simulink model "Model"  (R2021b)
settings: Solver=VariableStepAuto  StartTime=0.0  StopTime=10  RelTol=1e-3
undefined symbols (not defined in the file): A, Am, B, Bm, C, C2, Cm, D, D2, Dm, gamma, gammar, kr, kx, P
settings Model: Creator=Daniel  LastModifiedBy=Daniel

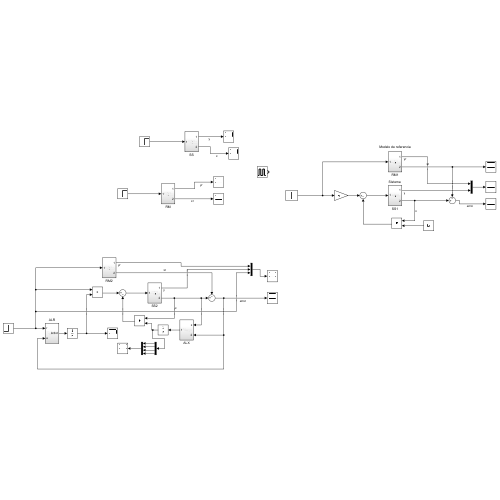
[thumbnail: Simulink's stored preview of the top-level diagram]
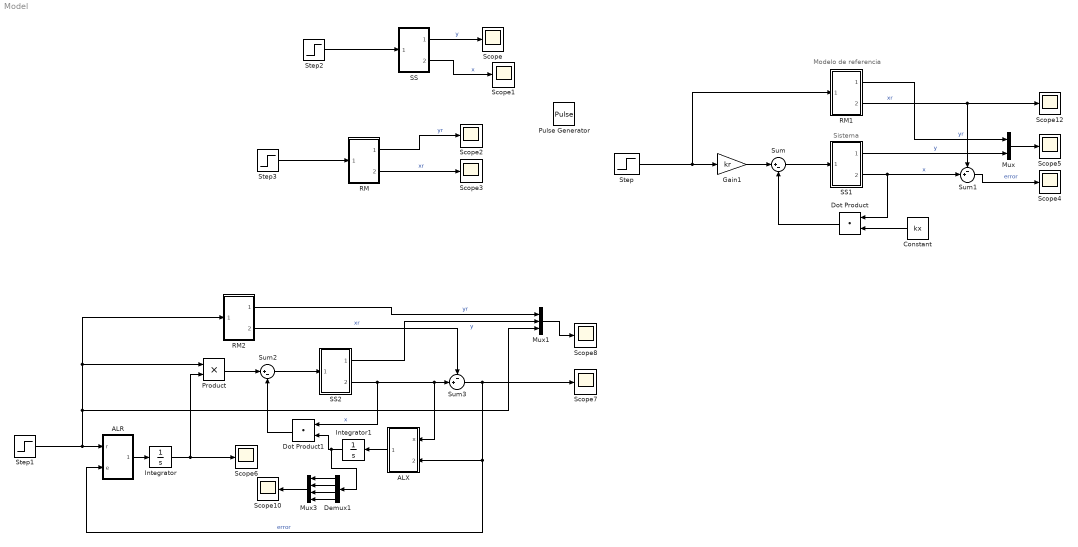
== system Model ==
  note: Sistema
  note: Modelo de referencia
  ALR : Subsystem
  ALX : Subsystem
  Constant : Constant  Value=kx
  Demux1 : Demux
  Dot Product : DotProduct  InputSameDT=on  OutDataTypeStr=Inherit: Inherit via internal rule
  Dot Product1 : DotProduct  InputSameDT=on  OutDataTypeStr=Inherit: Inherit via internal rule
  Gain1 : Gain  Gain=kr
  Integrator : Integrator  InitialCondition=kr
  Integrator1 : Integrator  InitialCondition=[kx]
  Mux : Mux  Inputs=2
  Mux1 : Mux  Inputs=3
  Mux3 : Mux
  Product : Product
  Pulse Generator : DiscretePulseGenerator  PulseType=Time based  Period=5  PulseWidth=50
  RM : Subsystem
  RM1 : Subsystem
  RM2 : Subsystem
  SS : Subsystem
  SS1 : Subsystem
  SS2 : Subsystem
  Scope{,1..8,10,12} (11 alike) : Scope
  Step : Step  Time=0  SampleTime=0
  Step1 : Step  SampleTime=0
  Step2 : Step  SampleTime=0
  Step3 : Step  Time=0  SampleTime=0
  Sum : Sum  Inputs=|+-
  Sum1 : Sum  Inputs=-+|
  Sum2 : Sum  Inputs=|+-
  Sum3 : Sum  Inputs=-+|
  wires:
  Step2/1 -> SS/1(In1)
  SS/1(Out1) -> Scope/1  "y"
  SS/2(Out2) -> Scope1/1  "x"
  Step3/1 -> RM/1(In1)
  RM/1(Out1) -> Scope2/1  "yr"
  RM/2(Out2) -> Scope3/1  "xr"
  SS1/2(Out2) -> Dot Product/1, Sum1/2  "x"
  Sum/1 -> SS1/1(In1)
  RM1/2(Out2) -> Scope12/1, Sum1/1  "xr"
  Dot Product/1 -> Sum/2
  Gain1/1 -> Sum/1
  Step/1 -> Gain1/1, RM1/1(In1)
  Sum1/1 -> Scope4/1  "error"
  Constant/1 -> Dot Product/2
  Sum3/1 -> Scope7/1, ALR/2(e), ALX/2(In2)  "error"
  Product/1 -> Sum2/1
  Dot Product1/1 -> Sum2/2
  RM2/2(Out2) -> Sum3/1  "xr"
  Sum2/1 -> SS2/1(In1)
  SS2/2(Out2) -> ALX/1(x), Sum3/2, Dot Product1/1  "x"
  ALR/1(krdot) -> Integrator/1
  Integrator/1 -> Scope6/1, Product/2
  ALX/1(Out1) -> Integrator1/1
  Integrator1/1 -> Demux1/1, Dot Product1/2
  Mux/1 -> Scope5/1
  RM1/1(Out1) -> Mux/1  "yr"
  SS1/1(Out1) -> Mux/2  "y"
  Step1/1 -> RM2/1(In1), Product/1, Mux1/3, ALR/1(r)
  RM2/1(Out1) -> Mux1/1  "yr"
  SS2/1(Out1) -> Mux1/2  "y"
  Mux1/1 -> Scope8/1
  Mux3/1 -> Scope10/1
  Demux1/1 -> Mux3/1
  Demux1/2 -> Mux3/2
  Demux1/3 -> Mux3/3
  Demux1/4 -> Mux3/4

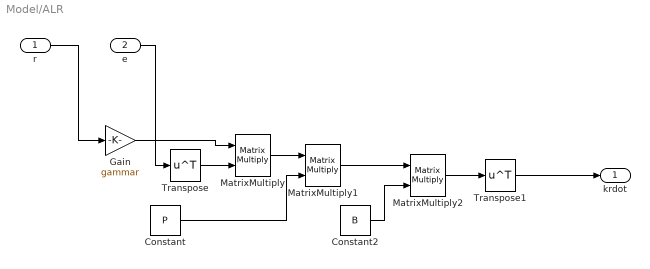
== system Model/ALR ==
  r : Inport
  e : Inport  Port=2
  Constant : Constant  Value=P
  Constant2 : Constant  Value=B
  Gain : Gain  Gain=gammar
  MatrixMultiply : Product  Multiplication=Matrix(*)
  MatrixMultiply1 : Product  Multiplication=Matrix(*)
  MatrixMultiply2 : Product  Multiplication=Matrix(*)
  Transpose : Math  Operator=transpose  SaturateOnIntegerOverflow=on
  Transpose1 : Math  Operator=transpose  SaturateOnIntegerOverflow=on
  krdot : Outport
  wires:
  Transpose1/1 -> krdot/1
  r/1 -> Gain/1
  e/1 -> Transpose/1
  MatrixMultiply1/1 -> MatrixMultiply2/1
  MatrixMultiply2/1 -> Transpose1/1
  Constant/1 -> MatrixMultiply1/2
  Constant2/1 -> MatrixMultiply2/2
  Gain/1 -> MatrixMultiply/1
  MatrixMultiply/1 -> MatrixMultiply1/1
  Transpose/1 -> MatrixMultiply/2

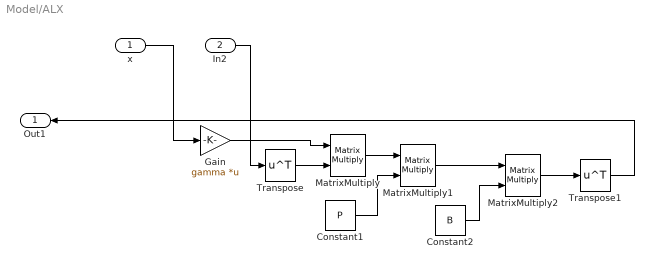
== system Model/ALX ==
  x : Inport
  In2 : Inport  Port=2
  Constant1 : Constant  Value=P
  Constant2 : Constant  Value=B
  Gain : Gain  Gain=gamma  Multiplication=Matrix(K*u)
  MatrixMultiply : Product  Multiplication=Matrix(*)
  MatrixMultiply1 : Product  Multiplication=Matrix(*)
  MatrixMultiply2 : Product  Multiplication=Matrix(*)
  Transpose : Math  Operator=transpose  SaturateOnIntegerOverflow=on
  Transpose1 : Math  Operator=transpose  SaturateOnIntegerOverflow=on
  Out1 : Outport
  wires:
  Transpose/1 -> MatrixMultiply/2
  MatrixMultiply/1 -> MatrixMultiply1/1
  Gain/1 -> MatrixMultiply/1
  Constant2/1 -> MatrixMultiply2/2
  Constant1/1 -> MatrixMultiply1/2
  MatrixMultiply2/1 -> Transpose1/1
  MatrixMultiply1/1 -> MatrixMultiply2/1
  In2/1 -> Transpose/1
  x/1 -> Gain/1
  Transpose1/1 -> Out1/1

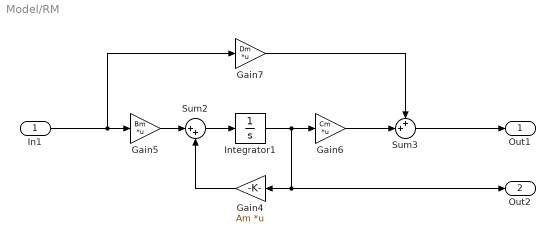
== system Model/RM ==
  In1 : Inport
  Gain4 : Gain  Gain=Am  Multiplication=Matrix(K*u)
  Gain5 : Gain  Gain=Bm  Multiplication=Matrix(K*u)
  Gain6 : Gain  Gain=Cm  Multiplication=Matrix(K*u)
  Gain7 : Gain  Gain=Dm  Multiplication=Matrix(K*u)
  Integrator1 : Integrator
  Sum2 : Sum  Inputs=|++
  Sum3 : Sum  Inputs=++|
  Out1 : Outport
  Out2 : Outport  Port=2
  wires:
  Sum3/1 -> Out1/1
  In1/1 -> Gain5/1, Gain7/1
  Integrator1/1 -> Gain6/1, Out2/1, Gain4/1
  Gain6/1 -> Sum3/2
  Gain7/1 -> Sum3/1
  Gain4/1 -> Sum2/2
  Gain5/1 -> Sum2/1
  Sum2/1 -> Integrator1/1

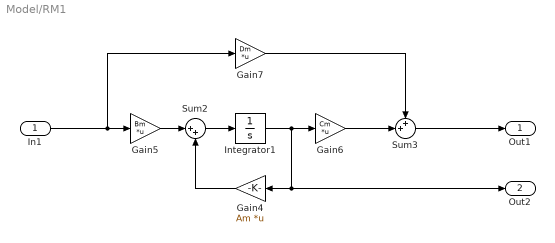
== system Model/RM1 ==
  In1 : Inport
  Gain4 : Gain  Gain=Am  Multiplication=Matrix(K*u)
  Gain5 : Gain  Gain=Bm  Multiplication=Matrix(K*u)
  Gain6 : Gain  Gain=Cm  Multiplication=Matrix(K*u)
  Gain7 : Gain  Gain=Dm  Multiplication=Matrix(K*u)
  Integrator1 : Integrator
  Sum2 : Sum  Inputs=|++
  Sum3 : Sum  Inputs=++|
  Out1 : Outport
  Out2 : Outport  Port=2
  wires:
  Sum2/1 -> Integrator1/1
  Gain5/1 -> Sum2/1
  Gain4/1 -> Sum2/2
  Gain7/1 -> Sum3/1
  Gain6/1 -> Sum3/2
  Integrator1/1 -> Gain4/1, Out2/1, Gain6/1
  In1/1 -> Gain7/1, Gain5/1
  Sum3/1 -> Out1/1

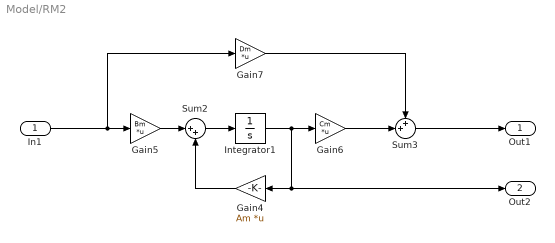
== system Model/RM2 ==
  In1 : Inport
  Gain4 : Gain  Gain=Am  Multiplication=Matrix(K*u)
  Gain5 : Gain  Gain=Bm  Multiplication=Matrix(K*u)
  Gain6 : Gain  Gain=Cm  Multiplication=Matrix(K*u)
  Gain7 : Gain  Gain=Dm  Multiplication=Matrix(K*u)
  Integrator1 : Integrator
  Sum2 : Sum  Inputs=|++
  Sum3 : Sum  Inputs=++|
  Out1 : Outport
  Out2 : Outport  Port=2
  wires:
  Sum3/1 -> Out1/1
  In1/1 -> Gain5/1, Gain7/1
  Integrator1/1 -> Gain6/1, Out2/1, Gain4/1
  Gain6/1 -> Sum3/2
  Gain7/1 -> Sum3/1
  Gain4/1 -> Sum2/2
  Gain5/1 -> Sum2/1
  Sum2/1 -> Integrator1/1

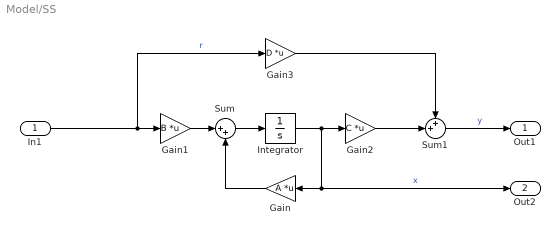
== system Model/SS ==
  In1 : Inport
  Gain : Gain  Gain=A  Multiplication=Matrix(K*u)
  Gain1 : Gain  Gain=B  Multiplication=Matrix(K*u)
  Gain2 : Gain  Gain=C  Multiplication=Matrix(K*u)
  Gain3 : Gain  Gain=D  Multiplication=Matrix(K*u)
  Integrator : Integrator
  Sum : Sum  Inputs=|++
  Sum1 : Sum  Inputs=++|
  Out1 : Outport
  Out2 : Outport  Port=2
  wires:
  Sum/1 -> Integrator/1
  In1/1 -> Gain3/1, Gain1/1  "r"
  Integrator/1 -> Out2/1, Gain/1, Gain2/1  "x"
  Gain3/1 -> Sum1/1
  Gain2/1 -> Sum1/2
  Gain1/1 -> Sum/1
  Sum1/1 -> Out1/1  "y"
  Gain/1 -> Sum/2

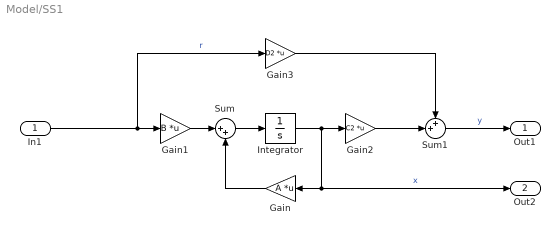
== system Model/SS1 ==
  In1 : Inport
  Gain : Gain  Gain=A  Multiplication=Matrix(K*u)
  Gain1 : Gain  Gain=B  Multiplication=Matrix(K*u)
  Gain2 : Gain  Gain=C2  Multiplication=Matrix(K*u)
  Gain3 : Gain  Gain=D2  Multiplication=Matrix(K*u)
  Integrator : Integrator
  Sum : Sum  Inputs=|++
  Sum1 : Sum  Inputs=++|
  Out1 : Outport
  Out2 : Outport  Port=2
  wires:
  Gain/1 -> Sum/2
  Sum1/1 -> Out1/1  "y"
  Gain1/1 -> Sum/1
  Gain2/1 -> Sum1/2
  Gain3/1 -> Sum1/1
  Integrator/1 -> Gain2/1, Gain/1, Out2/1  "x"
  In1/1 -> Gain1/1, Gain3/1  "r"
  Sum/1 -> Integrator/1

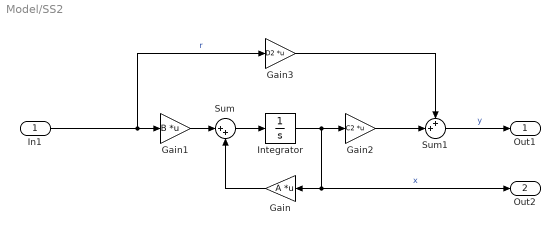
== system Model/SS2 ==
  In1 : Inport
  Gain : Gain  Gain=A  Multiplication=Matrix(K*u)
  Gain1 : Gain  Gain=B  Multiplication=Matrix(K*u)
  Gain2 : Gain  Gain=C2  Multiplication=Matrix(K*u)
  Gain3 : Gain  Gain=D2  Multiplication=Matrix(K*u)
  Integrator : Integrator
  Sum : Sum  Inputs=|++
  Sum1 : Sum  Inputs=++|
  Out1 : Outport
  Out2 : Outport  Port=2
  wires:
  Sum/1 -> Integrator/1
  In1/1 -> Gain3/1, Gain1/1  "r"
  Integrator/1 -> Out2/1, Gain/1, Gain2/1  "x"
  Gain3/1 -> Sum1/1
  Gain2/1 -> Sum1/2
  Gain1/1 -> Sum/1
  Sum1/1 -> Out1/1  "y"
  Gain/1 -> Sum/2
